simulink model "bpskModulation"  (R2021a)
settings: Solver=VariableStepAuto  StartTime=0.0  StopTime=10.0  RelTol=1e-3
libraries: visionsources x1
settings Model: Creator=manami  LastModifiedBy=manami

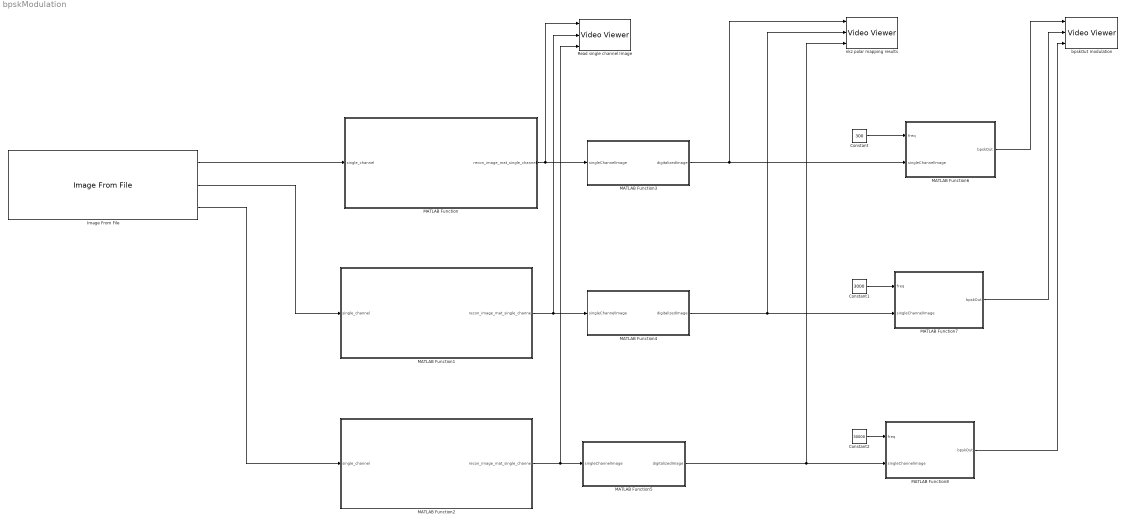
== system bpskModulation ==
  Constant : Constant  Value=300
  Constant1 : Constant  Value=3000
  Constant2 : Constant  Value=30000
  Image From File : visionsources/Image From File  Tag=vipblks_nd  FileName=D:\com project\174423899_808724736692372_8447064076947490794_n.jpg  Ts=inf  imagePorts=Separate color signals  OutPortLabels=R|G|B  ImageDataType=Inherit from input image  sdImageDataType=uint(8)  Signed=on  WordLength=16  FractionLengthMode=User-defined  FractionLength=15
  MATLAB Function : MATLAB Function  TreatAsAtomicUnit=on
  MATLAB Function1 : MATLAB Function  TreatAsAtomicUnit=on
  MATLAB Function2 : MATLAB Function  TreatAsAtomicUnit=on
  MATLAB Function3 : MATLAB Function  TreatAsAtomicUnit=on
  MATLAB Function4 : MATLAB Function  TreatAsAtomicUnit=on
  MATLAB Function5 : MATLAB Function  TreatAsAtomicUnit=on
  MATLAB Function6 : MATLAB Function  TreatAsAtomicUnit=on
  MATLAB Function7 : MATLAB Function  TreatAsAtomicUnit=on
  MATLAB Function8 : MATLAB Function  TreatAsAtomicUnit=on
  Read single channel Image : VideoViewer  imagePorts=separate color signals  FigPos=[1 1038 1920 938]
  bpskOut modulation : VideoViewer  imagePorts=separate color signals  FigPos=[1 1038 1920 938]
  nkz polar mapping results : VideoViewer  imagePorts=separate color signals  FigPos=[1 1038 1920 938]
  wires:
  MATLAB Function8/1(bpskOut) -> bpskOut modulation/3
  MATLAB Function5/1(digitalizedImage) -> MATLAB Function8/2(singleChannelImage), nkz polar mapping results/3
  MATLAB Function2/1(recon_image_mat_single_channel) -> MATLAB Function5/1(singleChannelImage), Read single channel Image/3
  MATLAB Function6/1(bpskOut) -> bpskOut modulation/1
  Constant/1 -> MATLAB Function6/1(freq)
  Image From File/3 -> MATLAB Function2/1(single_channel)
  MATLAB Function7/1(bpskOut) -> bpskOut modulation/2
  MATLAB Function4/1(digitalizedImage) -> MATLAB Function7/2(singleChannelImage), nkz polar mapping results/2
  Constant2/1 -> MATLAB Function8/1(freq)
  Constant1/1 -> MATLAB Function7/1(freq)
  MATLAB Function/1(recon_image_mat_single_channel) -> Read single channel Image/1, MATLAB Function3/1(singleChannelImage)
  MATLAB Function1/1(recon_image_mat_single_channel) -> MATLAB Function4/1(singleChannelImage), Read single channel Image/2
  Image From File/2 -> MATLAB Function1/1(single_channel)
  Image From File/1 -> MATLAB Function/1(single_channel)
  MATLAB Function3/1(digitalizedImage) -> MATLAB Function6/2(singleChannelImage), nkz polar mapping results/1

== matlab function bpskModulation/MATLAB Function ==
  data: single_channel input; recon_image_mat_single_channel output
function recon_image_mat_single_channel = single_channel_image_read(single_channel)
%#codegen
row = length(single_channel(:,1));
col = length(single_channel);
bin = zeros(1,row*col);;
k=1;
for i=1:row
    bin(1,k:k+col-1) = single_channel(i,:);
    k = k+col;
end
binla = dec2bin(bin);
bintemp = binla;
bintemp(:,7:8) = '0';
new = bin2dec(bintemp)';
recon = zeros(row,col);
for i = 1:row
    recon(i,1:col) = new(1,col*(i-1)+1:col*i);
end 
newimage = recon;
recon_image_mat_single_channel = cast(newimage,'uint8');

== matlab function bpskModulation/MATLAB Function2 ==
  data: single_channel input; recon_image_mat_single_channel output
function recon_image_mat_single_channel = single_channel_image_read(single_channel)
%#codegen
row = length(single_channel(:,1));
col = length(single_channel);
bin = zeros(1,row*col);;
k=1;
for i=1:row
    bin(1,k:k+col-1) = single_channel(i,:);
    k = k+col;
end
binla = dec2bin(bin);
bintemp = binla;
bintemp(:,7:8) = '0';
new = bin2dec(bintemp)';
recon = zeros(row,col);
for i = 1:row
    recon(i,1:col) = new(1,col*(i-1)+1:col*i);
end 
newimage = recon;
recon_image_mat_single_channel = cast(newimage,'uint8');

== matlab function bpskModulation/MATLAB Function3 ==
  data: singleChannelImage input; digitalizedImage output
function digitalizedImage = nkz_polar_mapping(singleChannelImage)
imageShape = size(singleChannelImage);
threshold = mean(singleChannelImage, 'all');
N = imageShape(2) % N = input size
% n = image row

% Unipolar mapping
for indImg = 1:imageShape(1)
    for i = 1:N
        if singleChannelImage(indImg, i)<=threshold
            singleChannelImage(indImg, i) = -1;
        else
            singleChannelImage(indImg, i) = 1;
        end          
    end
end
digitalizedImage = singleChannelImage;

%NOTE: we have used the mean pixel as threshold for unipolar mapping
%NOTE: I do not need the continuous assigning variable thing for now, if I
%this, the quality will be better, we will keep this for later
%NOTE: Single Channel Image Dim 1932*2576

== matlab function bpskModulation/MATLAB Function4 ==
  data: singleChannelImage input; digitalizedImage output
function digitalizedImage = nkz_polar_mapping(singleChannelImage)
imageShape = size(singleChannelImage);
threshold = mean(singleChannelImage, 'all');
N = imageShape(2) % N = input size
% n = image row

% Unipolar mapping
for indImg = 1:imageShape(1)
    for i = 1:N
        if singleChannelImage(indImg, i)<=threshold
            singleChannelImage(indImg, i) = -1;
        else
            singleChannelImage(indImg, i) = 1;
        end          
    end
end
digitalizedImage = singleChannelImage;

%NOTE: we have used the mean pixel as threshold for unipolar mapping
%NOTE: I do not need the continuous assigning variable thing for now, if I
%this, the quality will be better, we will keep this for later
%NOTE: Single Channel Image Dim 1932*2576

== matlab function bpskModulation/MATLAB Function5 ==
  data: singleChannelImage input; digitalizedImage output
function digitalizedImage = nkz_polar_mapping(singleChannelImage)
imageShape = size(singleChannelImage);
threshold = mean(singleChannelImage, 'all');
N = imageShape(2) % N = input size
% n = image row

% Unipolar mapping
for indImg = 1:imageShape(1)
    for i = 1:N
        if singleChannelImage(indImg, i)<=threshold
            singleChannelImage(indImg, i) = -1;
        else
            singleChannelImage(indImg, i) = 1;
        end          
    end
end
digitalizedImage = singleChannelImage;

%NOTE: we have used the mean pixel as threshold for unipolar mapping
%NOTE: I do not need the continuous assigning variable thing for now, if I
%this, the quality will be better, we will keep this for later
%NOTE: Single Channel Image Dim 1932*2576

== matlab function bpskModulation/MATLAB Function6 ==
  data: freq input; bpskOut output; singleChannelImage input
function bpskOut = bpsk_signal(freq, singleChannelImage)
sizeIm = size(singleChannelImage)
bpskOut = zeros(sizeIm)
carrier = cos(2*pi*freq*sizeIm(2))
% for i = 1: sizeIm(1)
%     baskOut(i, :) = singleChannelImage(i, :).*carrier
% end
bpskOut(:, :) = singleChannelImage.*carrier
bpskOut = bpskOut;

== matlab function bpskModulation/MATLAB Function7 ==
  data: freq input; bpskOut output; singleChannelImage input
function bpskOut = bpsk_signal(freq, singleChannelImage)
sizeIm = size(singleChannelImage)
bpskOut = zeros(sizeIm)
carrier = cos(2*pi*freq*sizeIm(2))
% for i = 1: sizeIm(1)
%     baskOut(i, :) = singleChannelImage(i, :).*carrier
% end
bpskOut(:, :) = singleChannelImage.*carrier
bpskOut = bpskOut;

== matlab function bpskModulation/MATLAB Function8 ==
  data: freq input; bpskOut output; singleChannelImage input
function bpskOut = bpsk_signal(freq, singleChannelImage)
sizeIm = size(singleChannelImage)
bpskOut = zeros(sizeIm)
carrier = cos(2*pi*freq*sizeIm(2))
% for i = 1: sizeIm(1)
%     baskOut(i, :) = singleChannelImage(i, :).*carrier
% end
bpskOut(:, :) = singleChannelImage.*carrier
bpskOut = bpskOut;

== matlab function bpskModulation/MATLAB Function1 ==
  data: single_channel input; recon_image_mat_single_channel output
function recon_image_mat_single_channel = single_channel_image_read(single_channel)
%#codegen
row = length(single_channel(:,1));
col = length(single_channel);
bin = zeros(1,row*col);;
k=1;
for i=1:row
    bin(1,k:k+col-1) = single_channel(i,:);
    k = k+col;
end
binla = dec2bin(bin);
bintemp = binla;
bintemp(:,7:8) = '0';
new = bin2dec(bintemp)';
recon = zeros(row,col);
for i = 1:row
    recon(i,1:col) = new(1,col*(i-1)+1:col*i);
end 
newimage = recon;
recon_image_mat_single_channel = cast(newimage,'uint8');
